simulink model "simLQG"  (R2020a)
settings: Solver=FixedStepAuto  StartTime=0.0  StopTime=0.25  FixedStep=1e-6  RelTol=1e-3
values from neighbouring files (symbols this model uses):
  A = blkdiag(Af, Aw)    [LQGdemo.m]    (also in LQGdemo2.m = blkdiag(A_sys, A_dist); LQRdemo.m = blkdiag(Af, A_w2))
  Af = [3.0413559308 1 0 0 0 0 0 0 -4.09943636845 0 1 0 ... (64 elements, 8x8)]    [systemIdentification.mat]
  Aw = [7.15731692377 1 0 0 0 0 0 0 -22.6330178373 0 1 0 ... (64 elements, 8x8)]    [bandlimitedNoise.mat]
  B = [Bf; zeros(p, size(Bf, 2))]    [LQGdemo.m]    (also in LQGdemo2.m = [B_sys; zeros(p, size(B_sys, 2))]; LQRdemo.m)
  Bf = [1 0 0 0 0 0 0 0]    [systemIdentification.mat]
  Bw = [1 0 0 0 0 0 0 0]    [bandlimitedNoise.mat]
  C = [Cf , Cw]    [LQGdemo.m]    (also in LQGdemo2.m = [C_sys, C_dist]; LQRdemo.m = [Cf , C_w2])
  Cf = [1.00003753161 -1.43234260286 0.481731109446 -1.28622000482 1.31363064627 -0.474439772874 1.42010597323 -1.02301085718]    [systemIdentification.mat]
  Cw = [0.0010315141178 -0.00383835649469 0.0059517005763 -0.00598848886077 0.0050995089237 -0.00297128749324 0.000649019459501 6.63882420652e-05]    [bandlimitedNoise.mat]
  Df = 0    [systemIdentification.mat]
  Dw = 0.000144120223932    [bandlimitedNoise.mat]
  K = lqg_controller.K    [LQGdemo2.m]
  L = lqg_controller.L    [LQGdemo2.m]
libraries: simulink x2
settings Model: Creator=胡子瀚  LastModifiedBy=胡子瀚
settings SolverCC: AlgebraicLoopSolver=LineSearch

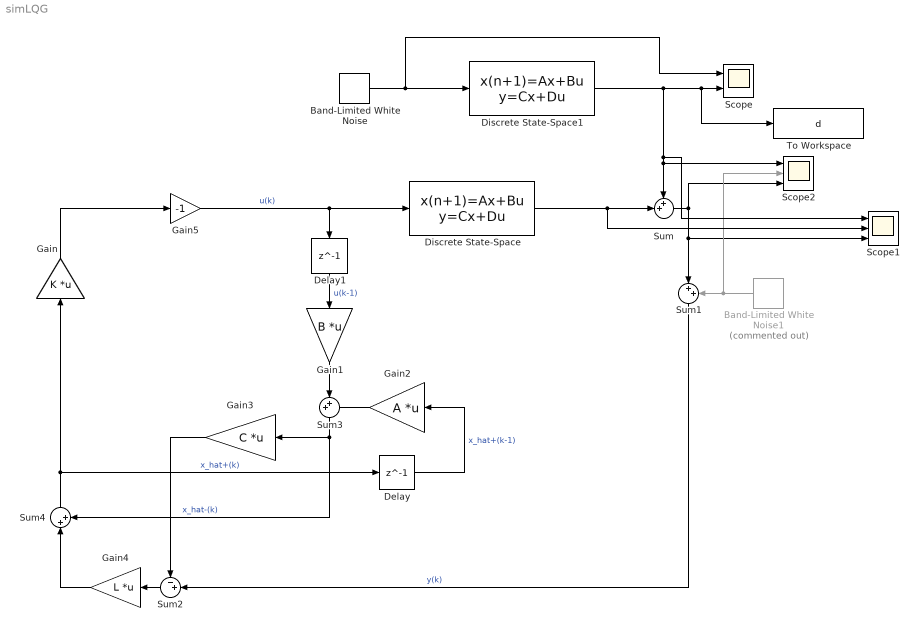
== system simLQG ==
  Band-Limited White Noise : simulink/Sources/Band-Limited White Noise  Cov=[0.002]  Ts=1.25e-4  seed=[23341]
  Band-Limited White Noise1 : simulink/Sources/Band-Limited White Noise  Commented=on  Cov=[0.001]  Ts=1.25e-4  seed=[23341]
  Delay : Delay  DelayLength=1
  Delay1 : Delay  DelayLength=1
  Discrete State-Space : DiscreteStateSpace  A=Af  B=Bf  C=Cf  D=Df  SampleTime=-1
  Discrete State-Space1 : DiscreteStateSpace  A=Aw  B=Bw  C=Cw  D=Dw  SampleTime=-1
  Gain : Gain  Gain=K  Multiplication=Matrix(K*u) (u vector)
  Gain1 : Gain  Gain=B  Multiplication=Matrix(K*u) (u vector)
  Gain2 : Gain  Gain=A  Multiplication=Matrix(K*u) (u vector)
  Gain3 : Gain  Gain=C  Multiplication=Matrix(K*u) (u vector)
  Gain4 : Gain  Gain=L  Multiplication=Matrix(K*u) (u vector)
  Gain5 : Gain  Gain=-1
  Scope : Scope  NumInputPorts=2
  Scope1 : Scope  NumInputPorts=3
  Scope2 : Scope  NumInputPorts=3
  Sum : Sum  Inputs=++|
  Sum1 : Sum  Inputs=|++
  Sum2 : Sum  Inputs=-+|
  Sum3 : Sum  Inputs=|++
  Sum4 : Sum  Inputs=|++
  To Workspace : ToWorkspace  VariableName=d  SampleTime=-1
  wires:
  Sum/1 -> Scope2/3, Scope1/3, Sum1/1
  Gain/1 -> Gain5/1
  Band-Limited White Noise1/1 -> Scope2/2, Sum1/2
  Gain1/1 -> Sum3/1
  Sum3/1 -> Sum4/2, Gain3/1  "x_hat-(k)"
  Delay/1 -> Gain2/1  "x_hat+(k-1)"
  Gain2/1 -> Sum3/2
  Sum1/1 -> Sum2/2  "y(k)"
  Gain3/1 -> Sum2/1
  Sum2/1 -> Gain4/1
  Sum4/1 -> Gain/1, Delay/1  "x_hat+(k)"
  Gain4/1 -> Sum4/1
  Gain5/1 -> Delay1/1, Discrete State-Space/1  "u(k)"
  Discrete State-Space/1 -> Scope1/2, Sum/2
  Discrete State-Space1/1 -> Scope1/1, Sum/1, Scope2/1, To Workspace/1, Scope/2
  Delay1/1 -> Gain1/1  "u(k-1)"
  Band-Limited White Noise/1 -> Scope/1, Discrete State-Space1/1
